simulink subsystem "Compute_Optitrack_Drone_TForms"  (R2024a)
settings: Solver=VariableStepAuto  StartTime=0.0  StopTime=10.0  RelTol=1e-3
libraries: robotcorelib x3
settings Model: Creator=Sasha  LastModifiedBy=Sasha

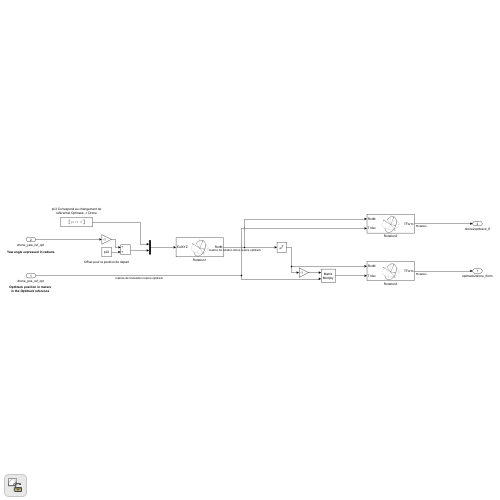
[thumbnail: Simulink's stored preview of the top-level diagram]
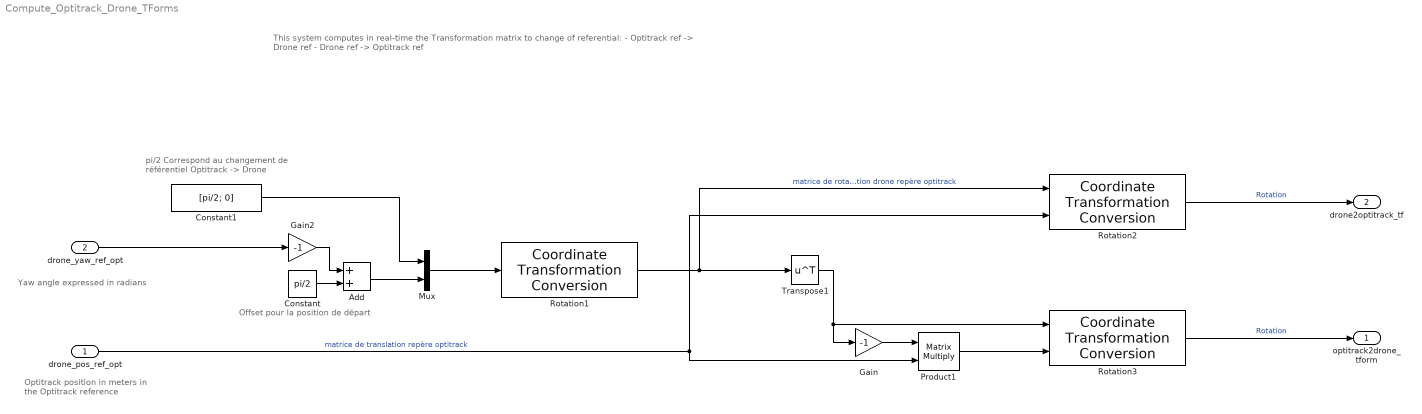
== system Compute_Optitrack_Drone_TForms ==
  note: This system computes in real-time the Transformation matrix to change of referential:
      | - Optitrack ref -> Drone ref
      | - Drone ref -> Optitrack ref
  note: Yaw angle expressed in radians
  note: Offset pour la position de départ
  note: pi/2 Correspond au changement de référentiel Optitrack -> Drone
  note: Optitrack position in meters
      | in the Optitrack reference
  drone_pos_ref_opt : Inport
  drone_yaw_ref_opt : Inport  Port=2
  Add : Sum
  Constant : Constant  Value=pi/2
  Constant1 : Constant  Value=[pi/2; 0]
  Gain : Gain  Gain=-1
  Gain2 : Gain  Gain=-1
  Mux : Mux  Inputs=2
  Product1 : Product  Multiplication=Matrix(*)
  Rotation1 : robotcorelib/Coordinate Transformation Conversion  InputRepresentation=Euler Angles  InputEulerSequence=XYZ  ShowTrVecInputPort=off  OutputRepresentation=Rotation Matrix  OutputEulerSequence=ZYX  ShowTrVecOutputPort=off  SimulateUsing=Code generation
      settings: LibrarySourceBlock=uavutilslib/Coordinate Transformation Conversion
  Rotation2 : robotcorelib/Coordinate Transformation Conversion  InputRepresentation=Rotation Matrix  InputEulerSequence=XYZ  ShowTrVecInputPort=on  OutputRepresentation=Homogeneous Transformation  OutputEulerSequence=ZYX  ShowTrVecOutputPort=off  SimulateUsing=Code generation
      settings: LibrarySourceBlock=uavutilslib/Coordinate Transformation Conversion
  Rotation3 : robotcorelib/Coordinate Transformation Conversion  InputRepresentation=Rotation Matrix  InputEulerSequence=XYZ  ShowTrVecInputPort=on  OutputRepresentation=Homogeneous Transformation  OutputEulerSequence=ZYX  ShowTrVecOutputPort=off  SimulateUsing=Code generation
      settings: LibrarySourceBlock=uavutilslib/Coordinate Transformation Conversion
  Transpose1 : Math  Operator=transpose
  optitrack2drone_tform : Outport
  drone2optitrack_tf : Outport  Port=2
  wires:
  Add/1 -> Mux/2
  Transpose1/1 -> Gain/1, Rotation3/1
  Constant/1 -> Add/2
  Gain2/1 -> Add/1
  Product1/1 -> Rotation3/2
  Constant1/1 -> Mux/1
  Rotation1/1 -> Transpose1/1, Rotation2/1  "matrice de rotation drone repère optitrack"
  Gain/1 -> Product1/1
  Mux/1 -> Rotation1/1
  drone_pos_ref_opt/1 -> Rotation2/2, Product1/2  "matrice de translation repère optitrack"
  drone_yaw_ref_opt/1 -> Gain2/1
  Rotation3/1 -> optitrack2drone_tform/1  "Rotation"
  Rotation2/1 -> drone2optitrack_tf/1  "Rotation"
